simulink model "PX4_Run_Mode_R2016b"  (R2017b)
settings: Solver=FixedStepDiscrete  StartTime=0.0  StopTime=inf  FixedStep=Ts  RelTol=1e-3  EnableMultiTasking=on
InitFcn:
  | run('InitFcn_R2016b.m');
values from neighbouring files (symbols this model uses):
  A = Pixhawk_CSC.Parameter( {single([diag([1 1 1]) Ts*diag([1 1 1]); diag([0 0 0]) diag([1 1 1])]),'A'} )    [InitFcn.m]    (also in InitFcn_R2016b.m; InitFcn_R2017b_no_csc.m = single([diag([1 1 1]) Ts*diag([1 1 1]); diag([0 0 0]) diag([)
  app = Pixhawk_CSC.Parameter({single( [0.05; 0.05; 0.05]),'app'} )    [InitFcn.m]    (also in InitFcn_R2016b.m; InitFcn_R2017b_no_csc.m = single( [0.05; 0.05; 0.05]))
  B = Pixhawk_CSC.Parameter( {single([Ts^2/2*diag([1 1 1]); Ts*diag([1 1 1])]),'B'} )    [InitFcn.m]    (also in InitFcn_R2016b.m; InitFcn_R2017b_no_csc.m = single([Ts^2/2*diag([1 1 1]); Ts*diag([1 1 1])]))
  Beta = Pixhawk_CSC.Parameter({single( 0.02),'Beta'} )    [InitFcn.m]    (also in InitFcn_R2016b.m; InitFcn_R2017b_no_csc.m = single( 0.02))
  C = Pixhawk_CSC.Parameter( {single([diag([1 1 1]) 0*diag([1 1 1]); zeros(1,2) 1 zeros(1,3)]),'C'} )    [InitFcn.m]    (also in InitFcn_R2016b.m; InitFcn_R2017b_no_csc.m = single([diag([1 1 1]) 0*diag([1 1 1]); zeros(1,2) 1 zeros(1,)
  C1 = Pixhawk_CSC.Parameter({single( 1.08680),'C1'} )    [InitFcn.m]    (also in InitFcn_R2016b.m; InitFcn_R2017b_no_csc.m = single( 1.08680))
  C10 = Pixhawk_CSC.Parameter({single( 0.0000),'C10'} )    [InitFcn.m]    (also in InitFcn_R2016b.m; InitFcn_R2017b_no_csc.m = single( 0.0000))
  C11 = Pixhawk_CSC.Parameter({single(-0.2300),'C11'} )    [InitFcn.m]    (also in InitFcn_R2016b.m; InitFcn_R2017b_no_csc.m = single(-0.2300))
  C12 = Pixhawk_CSC.Parameter({single( 0.0000),'C12'} )    [InitFcn.m]    (also in InitFcn_R2016b.m; InitFcn_R2017b_no_csc.m = single( 0.0000))
  C13 = Pixhawk_CSC.Parameter({single( 0.8000),'C13'} )    [InitFcn.m]    (also in InitFcn_R2016b.m; InitFcn_R2017b_no_csc.m = single( 0.8000))
  C14 = Pixhawk_CSC.Parameter({single( 0.8000),'C14'} )    [InitFcn.m]    (also in InitFcn_R2016b.m; InitFcn_R2017b_no_csc.m = single( 0.8000))
  C15 = Pixhawk_CSC.Parameter({single( 1.73200),'C15'} )    [InitFcn.m]    (also in InitFcn_R2016b.m; InitFcn_R2017b_no_csc.m = single( 1.73200))
  C16 = Pixhawk_CSC.Parameter({single( 0.1000),'C16'} )    [InitFcn.m]    (also in InitFcn_R2016b.m; InitFcn_R2017b_no_csc.m = single( 0.1000))
  C17 = Pixhawk_CSC.Parameter({single( 0.1000),'C17'} )    [InitFcn.m]    (also in InitFcn_R2016b.m; InitFcn_R2017b_no_csc.m = single( 0.1000))
  C18 = Pixhawk_CSC.Parameter({single( 0.0500),'C18'} )    [InitFcn.m]    (also in InitFcn_R2016b.m; InitFcn_R2017b_no_csc.m = single( 0.0500))
  C19 = Pixhawk_CSC.Parameter({single( 0.6000),'C19'} )    [InitFcn.m]    (also in InitFcn_R2016b.m; InitFcn_R2017b_no_csc.m = single( 0.6000))
  C2 = Pixhawk_CSC.Parameter({single( 1.10468),'C2'} )    [InitFcn.m]    (also in InitFcn_R2016b.m; InitFcn_R2017b_no_csc.m = single( 1.10468))
  C20 = Pixhawk_CSC.Parameter({single( 0.6000),'C20'} )    [InitFcn.m]    (also in InitFcn_R2016b.m; InitFcn_R2017b_no_csc.m = single( 0.6000))
  C21 = Pixhawk_CSC.Parameter({single( 1.04558),'C21'} )    [InitFcn.m]    (also in InitFcn_R2016b.m; InitFcn_R2017b_no_csc.m = single( 1.04558))
  C22 = Pixhawk_CSC.Parameter({single( 0.0000),'C22'} )    [InitFcn.m]    (also in InitFcn_R2016b.m; InitFcn_R2017b_no_csc.m = single( 0.0000))
  C23 = Pixhawk_CSC.Parameter({single( 0.0000),'C23'} )    [InitFcn.m]    (also in InitFcn_R2016b.m; InitFcn_R2017b_no_csc.m = single( 0.0000))
  C24 = Pixhawk_CSC.Parameter({single(-11.0000),'C24'} )    [InitFcn.m]    (also in InitFcn_R2016b.m; InitFcn_R2017b_no_csc.m = single(-11.0000))
  C3 = Pixhawk_CSC.Parameter({single( 1.1980),'C3'} )    [InitFcn.m]    (also in InitFcn_R2016b.m; InitFcn_R2017b_no_csc.m = single( 1.1980))
  C4 = Pixhawk_CSC.Parameter({single( 0.0500),'C4'} )    [InitFcn.m]    (also in InitFcn_R2016b.m; InitFcn_R2017b_no_csc.m = single( 0.0500))
  C5 = Pixhawk_CSC.Parameter({single( 0.0500),'C5'} )    [InitFcn.m]    (also in InitFcn_R2016b.m; InitFcn_R2017b_no_csc.m = single( 0.0500))
  C6 = Pixhawk_CSC.Parameter({single( 0.0500),'C6'} )    [InitFcn.m]    (also in InitFcn_R2016b.m; InitFcn_R2017b_no_csc.m = single( 0.0500))
  C7 = Pixhawk_CSC.Parameter({single( 0.35937),'C7'} )    [InitFcn.m]    (also in InitFcn_R2016b.m; InitFcn_R2017b_no_csc.m = single( 0.35937))
  C8 = Pixhawk_CSC.Parameter({single( 0.36528),'C8'} )    [InitFcn.m]    (also in InitFcn_R2016b.m; InitFcn_R2017b_no_csc.m = single( 0.36528))
  C9 = Pixhawk_CSC.Parameter({single( 0.53311),'C9'} )    [InitFcn.m]    (also in InitFcn_R2016b.m; InitFcn_R2017b_no_csc.m = single( 0.53311))
  C_1 = Pixhawk_CSC.Parameter( {single([diag([1 1 1]) 0*diag([1 1 1])]),'C1'} )    [InitFcn.m]    (also in InitFcn_R2016b.m; InitFcn_R2017b_no_csc.m = single([diag([1 1 1]) 0*diag([1 1 1])]))
  CAL_ACC0_XOFFSET = Pixhawk_CSC.Parameter( {single( 0.122052  ),'CAL_ACC0_XOFFSET'} )    [InitFcn.m]    (also in InitFcn_R2016b.m; InitFcn_R2017b_no_csc.m = single( 0.122052  ))
  CAL_ACC0_XXSCALE = Pixhawk_CSC.Parameter( {single(  1.01218    ),'CAL_ACC0_XXSCALE'} )    [InitFcn.m]    (also in InitFcn_R2016b.m; InitFcn_R2017b_no_csc.m = single(  1.01218    ))
  CAL_ACC0_XYSCALE = Pixhawk_CSC.Parameter( {single( -0.00443301 ),'CAL_ACC0_XYSCALE'} )    [InitFcn.m]    (also in InitFcn_R2016b.m; InitFcn_R2017b_no_csc.m = single( -0.00443301 ))
  CAL_ACC0_XZSCALE = Pixhawk_CSC.Parameter( {single( -0.00505793 ),'CAL_ACC0_XZSCALE'} )    [InitFcn.m]    (also in InitFcn_R2016b.m; InitFcn_R2017b_no_csc.m = single( -0.00505793 ))
  CAL_ACC0_YOFFSET = Pixhawk_CSC.Parameter( {single( 0.00281205),'CAL_ACC0_YOFFSET'} )    [InitFcn.m]    (also in InitFcn_R2016b.m; InitFcn_R2017b_no_csc.m = single( 0.00281205))
  CAL_ACC0_YXSCALE = Pixhawk_CSC.Parameter( {single( -0.00443301 ),'CAL_ACC0_YXSCALE'} )    [InitFcn.m]    (also in InitFcn_R2016b.m; InitFcn_R2017b_no_csc.m = single( -0.00443301 ))
  CAL_ACC0_YYSCALE = Pixhawk_CSC.Parameter( {single(  1.00234    ),'CAL_ACC0_YYSCALE'} )    [InitFcn.m]    (also in InitFcn_R2016b.m; InitFcn_R2017b_no_csc.m = single(  1.00234    ))
  CAL_ACC0_YZSCALE = Pixhawk_CSC.Parameter( {single(  0.0160883  ),'CAL_ACC0_YZSCALE'} )    [InitFcn.m]    (also in InitFcn_R2016b.m; InitFcn_R2017b_no_csc.m = single(  0.0160883  ))
  CAL_ACC0_ZOFFSET = Pixhawk_CSC.Parameter( {single(-0.0298121 ),'CAL_ACC0_ZOFFSET'} )    [InitFcn.m]    (also in InitFcn_R2016b.m; InitFcn_R2017b_no_csc.m = single(-0.0298121 ))
  CAL_ACC0_ZXSCALE = Pixhawk_CSC.Parameter( {single( -0.00505793 ),'CAL_ACC0_ZXSCALE'} )    [InitFcn.m]    (also in InitFcn_R2016b.m; InitFcn_R2017b_no_csc.m = single( -0.00505793 ))
  CAL_ACC0_ZYSCALE = Pixhawk_CSC.Parameter( {single(  0.0160883  ),'CAL_ACC0_ZYSCALE'} )    [InitFcn.m]    (also in InitFcn_R2016b.m; InitFcn_R2017b_no_csc.m = single(  0.0160883  ))
  CAL_ACC0_ZZSCALE = Pixhawk_CSC.Parameter( {single(  0.983604   ),'CAL_ACC0_ZZSCALE'} )    [InitFcn.m]    (also in InitFcn_R2016b.m; InitFcn_R2017b_no_csc.m = single(  0.983604   ))
  CAL_BAR_OFFSET = Pixhawk_CSC.Parameter( {single( -20.8468),'CAL_BAR_OFFSET'} )    [InitFcn.m]    (also in InitFcn_R2016b.m; InitFcn_R2017b_no_csc.m = single( -20.8468))
  CAL_BAR_SCALE = Pixhawk_CSC.Parameter( {single(   1.0632),'CAL_BAR_SCALE'} )    [InitFcn.m]    (also in InitFcn_R2016b.m; InitFcn_R2017b_no_csc.m = single(   1.0632))
  CAL_BAT0_XOFFSET = Pixhawk_CSC.Parameter( {single( 0.0000),'CAL_BAT0_XOFFSET'} )    [InitFcn.m]    (also in InitFcn_R2016b.m; InitFcn_R2017b_no_csc.m = single( 0.0000))
  CAL_BAT0_XXSCALE = Pixhawk_CSC.Parameter( {single(  1.0000),'CAL_BAT0_XXSCALE'} )    [InitFcn.m]    (also in InitFcn_R2016b.m; InitFcn_R2017b_no_csc.m = single(  1.0000))
  CAL_BAT0_XYSCALE = Pixhawk_CSC.Parameter( {single(  0.0000),'CAL_BAT0_XYSCALE'} )    [InitFcn.m]    (also in InitFcn_R2016b.m; InitFcn_R2017b_no_csc.m = single(  0.0000))
  CAL_BAT0_XZSCALE = Pixhawk_CSC.Parameter( {single(  0.0000),'CAL_BAT0_XZSCALE'} )    [InitFcn.m]    (also in InitFcn_R2016b.m; InitFcn_R2017b_no_csc.m = single(  0.0000))
  CAL_BAT0_YOFFSET = Pixhawk_CSC.Parameter( {single( 0.0000),'CAL_BAT0_YOFFSET'} )    [InitFcn.m]    (also in InitFcn_R2016b.m; InitFcn_R2017b_no_csc.m = single( 0.0000))
  CAL_BAT0_YXSCALE = Pixhawk_CSC.Parameter( {single(  0.0000),'CAL_BAT0_YXSCALE'} )    [InitFcn.m]    (also in InitFcn_R2016b.m; InitFcn_R2017b_no_csc.m = single(  0.0000))
  CAL_BAT0_YYSCALE = Pixhawk_CSC.Parameter( {single(  1.0000),'CAL_BAT0_YYSCALE'} )    [InitFcn.m]    (also in InitFcn_R2016b.m; InitFcn_R2017b_no_csc.m = single(  1.0000))
  CAL_BAT0_YZSCALE = Pixhawk_CSC.Parameter( {single(  0.0000),'CAL_BAT0_YZSCALE'} )    [InitFcn.m]    (also in InitFcn_R2016b.m; InitFcn_R2017b_no_csc.m = single(  0.0000))
  CAL_BAT0_ZOFFSET = Pixhawk_CSC.Parameter( {single( 0.0000),'CAL_BAT0_ZOFFSET'} )    [InitFcn.m]    (also in InitFcn_R2016b.m; InitFcn_R2017b_no_csc.m = single( 0.0000))
  CAL_BAT0_ZXSCALE = Pixhawk_CSC.Parameter( {single(  0.0000),'CAL_BAT0_ZXSCALE'} )    [InitFcn.m]    (also in InitFcn_R2016b.m; InitFcn_R2017b_no_csc.m = single(  0.0000))
  CAL_BAT0_ZYSCALE = Pixhawk_CSC.Parameter( {single(  0.0000),'CAL_BAT0_ZYSCALE'} )    [InitFcn.m]    (also in InitFcn_R2016b.m; InitFcn_R2017b_no_csc.m = single(  0.0000))
  CAL_BAT0_ZZSCALE = Pixhawk_CSC.Parameter( {single(  1.0000),'CAL_BAT0_ZZSCALE'} )    [InitFcn.m]    (also in InitFcn_R2016b.m; InitFcn_R2017b_no_csc.m = single(  1.0000))
  CAL_GPS0_XOFFSET = Pixhawk_CSC.Parameter( {single( 0.0000),'CAL_GPS0_XOFFSET'} )    [InitFcn.m]    (also in InitFcn_R2016b.m; InitFcn_R2017b_no_csc.m = single( 0.0000))
  CAL_GPS0_XXSCALE = Pixhawk_CSC.Parameter( {single(  0.0100),'CAL_GPS0_XXSCALE'} )    [InitFcn.m]    (also in InitFcn_R2016b.m; InitFcn_R2017b_no_csc.m = single(  0.0100))
  CAL_GPS0_XYSCALE = Pixhawk_CSC.Parameter( {single(  0.0000),'CAL_GPS0_XYSCALE'} )    [InitFcn.m]    (also in InitFcn_R2016b.m; InitFcn_R2017b_no_csc.m = single(  0.0000))
  CAL_GPS0_XZSCALE = Pixhawk_CSC.Parameter( {single(  0.0000),'CAL_GPS0_XZSCALE'} )    [InitFcn.m]    (also in InitFcn_R2016b.m; InitFcn_R2017b_no_csc.m = single(  0.0000))
  CAL_GPS0_YOFFSET = Pixhawk_CSC.Parameter( {single( 0.0000),'CAL_GPS0_YOFFSET'} )    [InitFcn.m]    (also in InitFcn_R2016b.m; InitFcn_R2017b_no_csc.m = single( 0.0000))
  CAL_GPS0_YXSCALE = Pixhawk_CSC.Parameter( {single(  0.0000),'CAL_GPS0_YXSCALE'} )    [InitFcn.m]    (also in InitFcn_R2016b.m; InitFcn_R2017b_no_csc.m = single(  0.0000))
  CAL_GPS0_YYSCALE = Pixhawk_CSC.Parameter( {single(  0.0100),'CAL_GPS0_YYSCALE'} )    [InitFcn.m]    (also in InitFcn_R2016b.m; InitFcn_R2017b_no_csc.m = single(  0.0100))
  CAL_GPS0_YZSCALE = Pixhawk_CSC.Parameter( {single(  0.0000),'CAL_GPS0_YZSCALE'} )    [InitFcn.m]    (also in InitFcn_R2016b.m; InitFcn_R2017b_no_csc.m = single(  0.0000))
  CAL_GPS0_ZOFFSET = Pixhawk_CSC.Parameter( {single( 0.0000),'CAL_GPS0_ZOFFSET'} )    [InitFcn.m]    (also in InitFcn_R2016b.m; InitFcn_R2017b_no_csc.m = single( 0.0000))
  CAL_GPS0_ZXSCALE = Pixhawk_CSC.Parameter( {single(  0.0000),'CAL_GPS0_ZXSCALE'} )    [InitFcn.m]    (also in InitFcn_R2016b.m; InitFcn_R2017b_no_csc.m = single(  0.0000))
  CAL_GPS0_ZYSCALE = Pixhawk_CSC.Parameter( {single(  0.0000),'CAL_GPS0_ZYSCALE'} )    [InitFcn.m]    (also in InitFcn_R2016b.m; InitFcn_R2017b_no_csc.m = single(  0.0000))
  CAL_GPS0_ZZSCALE = Pixhawk_CSC.Parameter( {single( -0.0010),'CAL_GPS0_ZZSCALE'} )    [InitFcn.m]    (also in InitFcn_R2016b.m; InitFcn_R2017b_no_csc.m = single( -0.0010))
  CAL_GYRO0_XXSCALE = Pixhawk_CSC.Parameter( {single(0.992736),'CAL_GYRO0_XXSCALE'} )    [InitFcn.m]    (also in InitFcn_R2016b.m; InitFcn_R2017b_no_csc.m = single(0.992736))
  CAL_GYRO0_XYSCALE = Pixhawk_CSC.Parameter( {single(0.0000),'CAL_GYRO0_XYSCALE'} )    [InitFcn.m]    (also in InitFcn_R2016b.m; InitFcn_R2017b_no_csc.m = single(0.0000))
  CAL_GYRO0_XZSCALE = Pixhawk_CSC.Parameter( {single(0.0000),'CAL_GYRO0_XZSCALE'} )    [InitFcn.m]    (also in InitFcn_R2016b.m; InitFcn_R2017b_no_csc.m = single(0.0000))
  CAL_GYRO0_YXSCALE = Pixhawk_CSC.Parameter( {single(0.0000),'CAL_GYRO0_YXSCALE'} )    [InitFcn.m]    (also in InitFcn_R2016b.m; InitFcn_R2017b_no_csc.m = single(0.0000))
  CAL_GYRO0_YYSCALE = Pixhawk_CSC.Parameter( {single(1.01609),'CAL_GYRO0_YYSCALE'} )    [InitFcn.m]    (also in InitFcn_R2016b.m; InitFcn_R2017b_no_csc.m = single(1.01609))
  CAL_GYRO0_YZSCALE = Pixhawk_CSC.Parameter( {single(0.0000),'CAL_GYRO0_YZSCALE'} )    [InitFcn.m]    (also in InitFcn_R2016b.m; InitFcn_R2017b_no_csc.m = single(0.0000))
  CAL_GYRO0_ZXSCALE = Pixhawk_CSC.Parameter( {single(0.0000),'CAL_GYRO0_ZXSCALE'} )    [InitFcn.m]    (also in InitFcn_R2016b.m; InitFcn_R2017b_no_csc.m = single(0.0000))
  CAL_GYRO0_ZYSCALE = Pixhawk_CSC.Parameter( {single(0.0000),'CAL_GYRO0_ZYSCALE'} )    [InitFcn.m]    (also in InitFcn_R2016b.m; InitFcn_R2017b_no_csc.m = single(0.0000))
  CAL_GYRO0_ZZSCALE = Pixhawk_CSC.Parameter( {single(1.03003),'CAL_GYRO0_ZZSCALE'} )    [InitFcn.m]    (also in InitFcn_R2016b.m; InitFcn_R2017b_no_csc.m = single(1.03003))
  CAL_MAG0_XCURCOR = Pixhawk_CSC.Parameter( {single( 0.0017     ),'CAL_MAG0_XCURCOR'} )    [InitFcn.m]    (also in InitFcn_R2016b.m; InitFcn_R2017b_no_csc.m = single( 0.0017     ))
  CAL_MAG0_XOFFSET = Pixhawk_CSC.Parameter( {single( 0.0446372  ),'CAL_MAG0_XOFFSET'} )    [InitFcn.m]    (also in InitFcn_R2016b.m; InitFcn_R2017b_no_csc.m = single( 0.0446372  ))
  CAL_MAG0_XXSCALE = Pixhawk_CSC.Parameter( {single(  1.01563   ),'CAL_MAG0_XXSCALE'} )    [InitFcn.m]    (also in InitFcn_R2016b.m; InitFcn_R2017b_no_csc.m = single(  1.01563   ))
  CAL_MAG0_XYSCALE = Pixhawk_CSC.Parameter( {single( -0.0612061 ),'CAL_MAG0_XYSCALE'} )    [InitFcn.m]    (also in InitFcn_R2016b.m; InitFcn_R2017b_no_csc.m = single( -0.0612061 ))
  CAL_MAG0_XZSCALE = Pixhawk_CSC.Parameter( {single( -0.011532  ),'CAL_MAG0_XZSCALE'} )    [InitFcn.m]    (also in InitFcn_R2016b.m; InitFcn_R2017b_no_csc.m = single( -0.011532  ))
  CAL_MAG0_YCURCOR = Pixhawk_CSC.Parameter( {single(-0.0075     ),'CAL_MAG0_YCURCOR'} )    [InitFcn.m]    (also in InitFcn_R2016b.m; InitFcn_R2017b_no_csc.m = single(-0.0075     ))
  CAL_MAG0_YOFFSET = Pixhawk_CSC.Parameter( {single( 0.0700776  ),'CAL_MAG0_YOFFSET'} )    [InitFcn.m]    (also in InitFcn_R2016b.m; InitFcn_R2017b_no_csc.m = single( 0.0700776  ))
  CAL_MAG0_YXSCALE = Pixhawk_CSC.Parameter( {single( -0.0612061 ),'CAL_MAG0_YXSCALE'} )    [InitFcn.m]    (also in InitFcn_R2016b.m; InitFcn_R2017b_no_csc.m = single( -0.0612061 ))
  CAL_MAG0_YYSCALE = Pixhawk_CSC.Parameter( {single(  1.00593   ),'CAL_MAG0_YYSCALE'} )    [InitFcn.m]    (also in InitFcn_R2016b.m; InitFcn_R2017b_no_csc.m = single(  1.00593   ))
  CAL_MAG0_YZSCALE = Pixhawk_CSC.Parameter( {single(  0.0144582 ),'CAL_MAG0_YZSCALE'} )    [InitFcn.m]    (also in InitFcn_R2016b.m; InitFcn_R2017b_no_csc.m = single(  0.0144582 ))
  CAL_MAG0_ZCURCOR = Pixhawk_CSC.Parameter( {single(-0.0080     ),'CAL_MAG0_ZCURCOR'} )    [InitFcn.m]    (also in InitFcn_R2016b.m; InitFcn_R2017b_no_csc.m = single(-0.0080     ))
  CAL_MAG0_ZOFFSET = Pixhawk_CSC.Parameter( {single( 0.00201742 ),'CAL_MAG0_ZOFFSET'} )    [InitFcn.m]    (also in InitFcn_R2016b.m; InitFcn_R2017b_no_csc.m = single( 0.00201742 ))
  CAL_MAG0_ZXSCALE = Pixhawk_CSC.Parameter( {single( -0.011532  ),'CAL_MAG0_ZXSCALE'} )    [InitFcn.m]    (also in InitFcn_R2016b.m; InitFcn_R2017b_no_csc.m = single( -0.011532  ))
  CAL_MAG0_ZYSCALE = Pixhawk_CSC.Parameter( {single(  0.0144582 ),'CAL_MAG0_ZYSCALE'} )    [InitFcn.m]    (also in InitFcn_R2016b.m; InitFcn_R2017b_no_csc.m = single(  0.0144582 ))
  CAL_MAG0_ZZSCALE = Pixhawk_CSC.Parameter( {single(  0.986813  ),'CAL_MAG0_ZZSCALE'} )    [InitFcn.m]    (also in InitFcn_R2016b.m; InitFcn_R2017b_no_csc.m = single(  0.986813  ))
  CAL_SONAR_OFFSET = Pixhawk_CSC.Parameter( {single( -6.8730),'CAL_SONAR_OFFSET'} )    [InitFcn.m]    (also in InitFcn_R2016b.m; InitFcn_R2017b_no_csc.m = single( -6.8730))
  CAL_SONAR_SCALE = Pixhawk_CSC.Parameter( {single(-438.1875),'CAL_SONAR_SCALE'} )    [InitFcn.m]    (also in InitFcn_R2016b.m; InitFcn_R2017b_no_csc.m = single(-438.1875))
  COM_RATE = double(10)    [InitFcn.m]    (also in InitFcn_R2016b.m; InitFcn_R2017b_no_csc.m)
  D = Pixhawk_CSC.Parameter( {single(zeros(size(C.Value,1), size(B.Value,2))),'D'} )    [InitFcn.m]    (also in InitFcn_R2016b.m; InitFcn_R2017b_no_csc.m = single(zeros(size(C,1), size(B,2))))
  Dip0 = Pixhawk_CSC.Parameter({single( 1.2),'Dip0'} )    [InitFcn.m]    (also in InitFcn_R2016b.m; InitFcn_R2017b_no_csc.m = single( 1.2))
  I = Pixhawk_CSC.Parameter( {single(eye(size(Q.Value))),'I'} )    [InitFcn.m]    (also in InitFcn_R2016b.m; InitFcn_R2017b_no_csc.m = single(eye(size(Q))))
  Jxx = Pixhawk_CSC.Parameter( {single(J(1,1)),'Jxx'} )    [InitFcn.m]    (also in InitFcn_R2016b.m; InitFcn_R2017b_no_csc.m = single(J(1,1)))
  Jyy = Pixhawk_CSC.Parameter( {single(J(2,2)),'Jyy'} )    [InitFcn.m]    (also in InitFcn_R2016b.m; InitFcn_R2017b_no_csc.m = single(J(2,2)))
  Jzz = Pixhawk_CSC.Parameter( {single(J(3,3)),'Jzz'} )    [InitFcn.m]    (also in InitFcn_R2016b.m; InitFcn_R2017b_no_csc.m = single(J(3,3)))
  Kapp = Pixhawk_CSC.Parameter({single( 1.2),'Kapp'} )    [InitFcn.m]    (also in InitFcn_R2016b.m; InitFcn_R2017b_no_csc.m = single( 1.2))
  Kx = Pixhawk_CSC.Parameter({single( Kx),'Kx'} )    [InitFcn.m]    (also in InitFcn_R2016b.m = Pixhawk_CSC.Parameter({single( [0.60 0.9]),'Kx'} ); InitFcn_R2017b_no_csc.m = single( [0.60 0.9]))
  Ky = Pixhawk_CSC.Parameter({single( Ky),'Ky'} )    [InitFcn.m]    (also in InitFcn_R2016b.m = Pixhawk_CSC.Parameter({single( [0.4 0.9]),'Ky'} ); InitFcn_R2017b_no_csc.m = single( [0.4 0.9]))
  LPF_REF_DEN = Pixhawk_CSC.Parameter( {single([1.0000 -0.8187]),'LPF_REF_DEN'} )    [InitFcn.m]    (also in InitFcn_R2016b.m; InitFcn_R2017b_no_csc.m = single([1.0000 -0.8187]))
  LPF_REF_NUM = Pixhawk_CSC.Parameter( {single([0.0000  0.1813]),'LPF_REF_NUM'} )    [InitFcn.m]    (also in InitFcn_R2016b.m; InitFcn_R2017b_no_csc.m = single([0.0000  0.1813]))
  m0 = Pixhawk_CSC.Parameter({single( 0.452857),'m0'} )    [InitFcn.m]    (also in InitFcn_R2016b.m; InitFcn_R2017b_no_csc.m = single( 0.452857))
  mn = [0.01; 0.01; 0.01; 0.01]    [InitFcn.m]    (also in InitFcn_R2016b.m; InitFcn_R2017b_no_csc.m)
  MOV_AVG_WINDOW = Pixhawk_CSC.Parameter( {single(100),'MOV_AVG_WINDOW'} )    [InitFcn.m]    (also in InitFcn_R2016b.m; InitFcn_R2017b_no_csc.m = single(100))
  Ox0 = Pixhawk_CSC.Parameter({single(O_x0),'Ox0'} )    [InitFcn.m]    (also in InitFcn_R2016b.m; InitFcn_R2017b_no_csc.m = single(O_x0))
  Oxa = Pixhawk_CSC.Parameter({single(O_x.a),'Oxa'} )    [InitFcn.m]    (also in InitFcn_R2016b.m; InitFcn_R2017b_no_csc.m = single(O_x.a))
  Oxb = Pixhawk_CSC.Parameter({single(O_x.b),'Oxb'} )    [InitFcn.m]    (also in InitFcn_R2016b.m; InitFcn_R2017b_no_csc.m = single(O_x.b))
  Oxc = Pixhawk_CSC.Parameter({single(O_x.c),'Oxc'} )    [InitFcn.m]    (also in InitFcn_R2016b.m; InitFcn_R2017b_no_csc.m = single(O_x.c))
  Oxd = Pixhawk_CSC.Parameter({single(O_x.d),'Oxd'} )    [InitFcn.m]    (also in InitFcn_R2016b.m; InitFcn_R2017b_no_csc.m = single(O_x.d))
  Oy0 = Pixhawk_CSC.Parameter({single(O_y0),'Oy0'} )    [InitFcn.m]    (also in InitFcn_R2016b.m; InitFcn_R2017b_no_csc.m = single(O_y0))
  Oya = Pixhawk_CSC.Parameter({single(O_y.a),'Oya'} )    [InitFcn.m]    (also in InitFcn_R2016b.m; InitFcn_R2017b_no_csc.m = single(O_y.a))
  Oyb = Pixhawk_CSC.Parameter({single(O_y.b),'Oyb'} )    [InitFcn.m]    (also in InitFcn_R2016b.m; InitFcn_R2017b_no_csc.m = single(O_y.b))
  Oyc = Pixhawk_CSC.Parameter({single(O_y.c),'Oyc'} )    [InitFcn.m]    (also in InitFcn_R2016b.m; InitFcn_R2017b_no_csc.m = single(O_y.c))
  Oyd = Pixhawk_CSC.Parameter({single(O_y.d),'Oyd'} )    [InitFcn.m]    (also in InitFcn_R2016b.m; InitFcn_R2017b_no_csc.m = single(O_y.d))
  Oz0 = Pixhawk_CSC.Parameter({single(O_z0),'Oz0'} )    [InitFcn.m]    (also in InitFcn_R2016b.m; InitFcn_R2017b_no_csc.m = single(O_z0))
  ... (+53 more)
undefined symbols (not defined in the file or in its folder): AccX, AccY, AccZ, Altitude, ax, ay, az, Current, FILTER_N, GPS_TS, GyroX, GyroY, GyroZ, Latitude, Longitude, M1_PWM, M2_PWM, M3_PWM, M4_PWM, MagX, MagY, MagZ, mAH, MOTOR, phi, Position_TS, psi, PX4_TUNE_ENUM, RGBLED_COLOR_ENUM, RGBLED_MODE_ENUM, S_AccX, S_AccY, S_AccZ, S_Altitude, S_Baro, S_Current, S_GyroX, S_GyroY, S_GyroZ, S_Latitude, S_Longitude, S_MagX, S_MagY, S_MagZ, S_mAH, S_N_Sat, S_Voltage, T_PITCH, T_ROLL, T_THROTTLE, theta, v, Voltage, w, wx, wxd, wy, wyd, wz ... (+4)
libraries: simulink x31, pixhawk_slib_sensors_actuators x7, pixhawk_slib_ADC_serial x5, pixhawk_slib_misc_utils x3, etargetslib x2
(part 3 of 7)

== system PX4_Run_Mode_R2016b/SENSOR_FILTER/Bias Removal State ==
  ESTIMATED_STATE_IN : Inport
  PARAMETERS_IN : Inport  Port=2
  SYSTEM_MODE_IN : Inport  Port=3
  Bus Assignment1 : BusAssignment  AssignedSignals=State Bias Parameters.X_BIAS,State Bias Parameters.Y_BIAS,State Bias Parameters.Z_BIAS,State Bias Parameters.PHI_BIAS,State Bias Parameters.THETA_BIAS,State Bias Parameters.PSI_BIAS,State Bias Parameters.U_BIAS,State Bias Parameters.V_BIAS,State Bias Parameters.W_BIAS,State Bias Parameters.WX_BIAS,State Bias Parameters.WY_BIAS,State Bias Parameters.WZ_BIAS,State Bias Parameters.AX_BIAS,State Bias Parameters.AY_BIAS,State Bias Parameters.AZ_BIAS,State Bias Parameters.WXD_BIAS,State Bias Parameters.WYD_BIAS,State Bias Parameters.WZD_BIAS
  Bus Assignment2 : BusAssignment  AssignedSignals=x,y,z,phi,theta,psi,u,v,w,wx,wy,wz,ax,ay,az,wxd,wyd,wzd
  Bus Selector1 : BusSelector  OutputSignals=ARM_CMD,PRE_ARM_CMD
  Bus Selector4 : BusSelector  OutputSignals=x,y,z,phi,theta,psi,u,v,w,wx,wy,wz,ax,ay,az,wxd,wyd,wzd  OutputAsBus=on
  Bus to Vector : BusToVector
  Demux1 : Demux  Outputs=18
  Demux2 : Demux  Outputs=18
  Logical Operator1 : Logic  IconShape=distinctive  AllPortsSameDT=off  OutDataTypeStr=boolean
  Logical Operator2 : Logic  Operator=NOT  IconShape=distinctive  AllPortsSameDT=off  OutDataTypeStr=boolean
  Logical Operator4 : Logic  Operator=NOT  IconShape=distinctive  AllPortsSameDT=off  OutDataTypeStr=boolean
  Logical Operator5 : Logic  IconShape=distinctive  AllPortsSameDT=off  OutDataTypeStr=boolean
  MATLAB Function3 : MATLAB Function  TreatAsAtomicUnit=on
  ESTIMATED_STATE_OUT : Outport
  PARAMETERS_OUT : Outport  Port=2
  wires:
  Bus to Vector/1 -> MATLAB Function3/1(STATE_IN)
  Bus Assignment2/1 -> ESTIMATED_STATE_OUT/1
  MATLAB Function3/1(STATE_OUT) -> Demux1/1
  ESTIMATED_STATE_IN/1 -> Bus Selector4/1, Bus Assignment2/1
  Bus Selector4/1 -> Bus to Vector/1
  SYSTEM_MODE_IN/1 -> Bus Selector1/1
  Bus Selector1/1 -> Logical Operator2/1  "<ARM_CMD>"
  Logical Operator2/1 -> Logical Operator1/1, Logical Operator5/1
  Bus Selector1/2 -> Logical Operator1/2, Logical Operator4/1  "<PRE_ARM_CMD>"
  Logical Operator5/1 -> MATLAB Function3/2(RESET)
  Logical Operator4/1 -> Logical Operator5/2
  Demux1/2 -> Bus Assignment2/3
  Demux1/1 -> Bus Assignment2/2
  Demux1/3 -> Bus Assignment2/4
  Demux1/7 -> Bus Assignment2/8
  Demux1/8 -> Bus Assignment2/9
  Demux1/9 -> Bus Assignment2/10
  Demux1/10 -> Bus Assignment2/11
  Demux1/11 -> Bus Assignment2/12
  Demux1/12 -> Bus Assignment2/13
  Demux1/13 -> Bus Assignment2/14
  Demux1/14 -> Bus Assignment2/15
  Demux1/15 -> Bus Assignment2/16
  Demux1/16 -> Bus Assignment2/17
  Demux1/17 -> Bus Assignment2/18
  Demux1/18 -> Bus Assignment2/19
  MATLAB Function3/2(BIAS_STATE) -> Demux2/1
  Demux2/18 -> Bus Assignment1/19
  Demux2/17 -> Bus Assignment1/18
  Demux2/16 -> Bus Assignment1/17
  Demux2/15 -> Bus Assignment1/16
  Demux2/14 -> Bus Assignment1/15
  Demux2/13 -> Bus Assignment1/14
  Demux2/12 -> Bus Assignment1/13
  Demux2/11 -> Bus Assignment1/12
  Demux2/10 -> Bus Assignment1/11
  Demux2/9 -> Bus Assignment1/10
  Demux2/8 -> Bus Assignment1/9
  Demux2/7 -> Bus Assignment1/8
  Demux2/6 -> Bus Assignment1/7
  Demux2/5 -> Bus Assignment1/6
  Demux2/3 -> Bus Assignment1/4
  Demux2/2 -> Bus Assignment1/3
  Demux2/4 -> Bus Assignment1/5
  Demux2/1 -> Bus Assignment1/2
  PARAMETERS_IN/1 -> Bus Assignment1/1
  Bus Assignment1/1 -> PARAMETERS_OUT/1
  Logical Operator1/1 -> MATLAB Function3/3(CONFIG_CMD)
  Demux1/4 -> Bus Assignment2/5
  Demux1/5 -> Bus Assignment2/6
  Demux1/6 -> Bus Assignment2/7

== system PX4_Run_Mode_R2016b/SENSOR_FILTER/Fixed Bias removal and scaling ==
  FILTERED_SENSOR_DATA_IN : Inport
  RAW_SENSOR_DATA_IN : Inport  Port=2
  SYSTEM_MODE_IN : Inport  Port=3
  Accelerometer Calibration : Subsystem
  Barometer Calibration : Subsystem
  Battery Calibration : Subsystem
  GPS Calibration : Subsystem
  Gyroscope Calibration : Subsystem
  MagnetoMeter Calibration : Subsystem
  Parameter Bus Creation : Subsystem
  Sonar Calibration : Subsystem
  FILTERED_SENSOR_DATA_OUT : Outport
  PARAMETERS_OUT : Outport  Port=2
  wires:
  RAW_SENSOR_DATA_IN/1 -> MagnetoMeter Calibration/2(RAW_SENSOR_DATA_IN), Accelerometer Calibration/2(RAW_SENSOR_DATA_IN), Gyroscope Calibration/2(RAW_SENSOR_DATA_IN), Barometer Calibration/2(RAW_SENSOR_DATA_IN), GPS Calibration/2(RAW_SENSOR_DATA_IN), Sonar Calibration/2(RAW_SENSOR_DATA_IN), Battery Calibration/2(RAW_SENSOR_DATA_IN)
  FILTERED_SENSOR_DATA_IN/1 -> MagnetoMeter Calibration/1(FILTERED_SENSOR_DATA_IN)
  MagnetoMeter Calibration/2(FILTERED_SENSOR_DATA_OUT) -> Accelerometer Calibration/1(FILTERED_SENSOR_DATA_IN)
  Accelerometer Calibration/2(FILTERED_SENSOR_DATA_OUT) -> Gyroscope Calibration/1(FILTERED_SENSOR_DATA_IN)
  SYSTEM_MODE_IN/1 -> GPS Calibration/3(SYSTEM_MODE_IN), Gyroscope Calibration/3(SYSTEM_MODE_IN)
  Gyroscope Calibration/2(FILTERED_SENSOR_DATA_OUT) -> Barometer Calibration/1(FILTERED_SENSOR_DATA_IN)
  GPS Calibration/2(FILTERED_SENSOR_DATA_OUT) -> Battery Calibration/1(FILTERED_SENSOR_DATA_IN)
  Battery Calibration/2(FILTERED_SENSOR_DATA_OUT) -> Sonar Calibration/1(FILTERED_SENSOR_DATA_IN)
  MagnetoMeter Calibration/1(Parameters) -> Parameter Bus Creation/1(Parameters Magnetometer)
  Accelerometer Calibration/1(Parameters) -> Parameter Bus Creation/2(Parameters Accelerometer)
  Gyroscope Calibration/1(Parameters) -> Parameter Bus Creation/3(Parameters Gyroscope)
  GPS Calibration/1(Parameters) -> Parameter Bus Creation/5(Parameters GPS)
  Battery Calibration/1(Parameters) -> Parameter Bus Creation/6(Parameters Battery)
  Parameter Bus Creation/1(Parameters) -> PARAMETERS_OUT/1
  Sonar Calibration/2(FILTERED_SENSOR_DATA_OUT) -> FILTERED_SENSOR_DATA_OUT/1
  Sonar Calibration/1(Parameters) -> Parameter Bus Creation/7(Parameters Sonar)
  Barometer Calibration/2(FILTERED_SENSOR_DATA_OUT) -> GPS Calibration/1(FILTERED_SENSOR_DATA_IN)
  Barometer Calibration/1(Parameters) -> Parameter Bus Creation/4(Parameters Barometer)

== system PX4_Run_Mode_R2016b/SENSOR_FILTER/SensorData2States ==
  ESTIMATED_STATE_IN : Inport
  FILTERED_SENSOR_DATA_IN : Inport  Port=2
  SYSTEM_MODE : Inport  Port=3
  Rotational State Estimation : Subsystem
  Translational State Estimation : Subsystem
  ESTIMATED_STATE_OUT : Outport
  wires:
  ESTIMATED_STATE_IN/1 -> Rotational State Estimation/2(ESTIMATED_STATE_IN)
  Translational State Estimation/1(ESTIMATED_STATE_OUT) -> ESTIMATED_STATE_OUT/1
  SYSTEM_MODE/1 -> Rotational State Estimation/1(SYSTEM_MODE_IN)
  FILTERED_SENSOR_DATA_IN/1 -> Translational State Estimation/2(FILTERED_SENSOR_DATA_IN), Rotational State Estimation/3(FILTERED_SENSOR_DATA_IN)
  Rotational State Estimation/1(ESTIMATED_STATE_OUT) -> Translational State Estimation/1(ESTIMATED_STATE_IN)

== system PX4_Run_Mode_R2016b/SENSOR_FILTER/StateEstimatesInitialConditions ==
  Bus Creator : BusCreator  Inputs=18
  Bus Creator1 : BusCreator  Inputs=18
  Demux : Demux  Outputs=18
  Demux1 : Demux  Outputs=18
  Initial_Filteres_Sensor_Data : MATLAB Function  TreatAsAtomicUnit=on
  State Estimater Initial Conditions : MATLAB Function  TreatAsAtomicUnit=on
  ESTIMATED_STATE_OUT : Outport
  FILTERED_SENSOR_DATA_OUT : Outport  Port=2
  wires:
  State Estimater Initial Conditions/1(Xhat) -> Demux/1
  Demux/6 -> Bus Creator/6  "psi"
  Demux/7 -> Bus Creator/7  "u"
  Demux/5 -> Bus Creator/5  "theta"
  Demux/4 -> Bus Creator/4  "phi"
  Demux/8 -> Bus Creator/8  "v"
  Demux/3 -> Bus Creator/3  "z"
  Demux/9 -> Bus Creator/9  "w"
  Demux/2 -> Bus Creator/2  "y"
  Demux/10 -> Bus Creator/10  "wx"
  Demux/1 -> Bus Creator/1  "x"
  Demux/11 -> Bus Creator/11  "wy"
  Demux/12 -> Bus Creator/12  "wz"
  Bus Creator/1 -> ESTIMATED_STATE_OUT/1
  Demux/13 -> Bus Creator/13  "ax"
  Demux/14 -> Bus Creator/14  "ay"
  Demux/15 -> Bus Creator/15  "az"
  Demux/16 -> Bus Creator/16  "wxd"
  Demux/17 -> Bus Creator/17  "wyd"
  Demux/18 -> Bus Creator/18  "wzd"
  Initial_Filteres_Sensor_Data/1(S) -> Demux1/1
  Bus Creator1/1 -> FILTERED_SENSOR_DATA_OUT/1
  Demux1/8 -> Bus Creator1/8  "GyroY"
  Demux1/7 -> Bus Creator1/7  "GyroX"
  Demux1/9 -> Bus Creator1/9  "GyroZ"
  Demux1/6 -> Bus Creator1/6  "AccZ"
  Demux1/10 -> Bus Creator1/10  "Bar"
  Demux1/11 -> Bus Creator1/11  "Latitude"
  Demux1/5 -> Bus Creator1/5  "AccY"
  Demux1/4 -> Bus Creator1/4  "AccX"
  Demux1/12 -> Bus Creator1/12  "Longitude"
  Demux1/13 -> Bus Creator1/13  "Altitude"
  Demux1/3 -> Bus Creator1/3  "MagZ"
  Demux1/2 -> Bus Creator1/2  "MagY"
  Demux1/14 -> Bus Creator1/14  "Num_Sat"
  Demux1/15 -> Bus Creator1/15  "Voltage"
  Demux1/1 -> Bus Creator1/1  "MagX"
  Demux1/16 -> Bus Creator1/16  "Current"
  Demux1/17 -> Bus Creator1/17  "mAH"
  Demux1/18 -> Bus Creator1/18  "Sonar"

== system PX4_Run_Mode_R2016b/CONTROLLER/Inner Control Loop/Pitch Control ==
  ERROR_IN : Inport
  TARGET : Inport  Port=2
  ESTIMATED_STATE_IN : Inport  Port=3
  "SYSTEM_MODE_IN " : Inport  Port=4
  Add1 : Sum  Inputs=+-
  Add3 : Sum  Inputs=+-
  Add4 : Sum  Inputs=++++
  Bus Assignment : BusAssignment  AssignedSignals=e6,e7,e8,e9,e10
  Bus Selector1 : BusSelector  OutputSignals=ARM_CMD
  Bus Selector10 : BusSelector  OutputSignals=T_PITCH
  Bus Selector11 : BusSelector  OutputSignals=theta,wy
  Constant : Constant  Value=0  SampleTime=Ts
  Constant1 : Constant  Value=C11  SampleTime=Ts
  Data Type Conversion : DataTypeConversion  OutDataTypeStr=single
  Gain : Gain  Gain=C2
  Gain1 : Gain  Gain=C8
  Logical Operator8 : Logic  Operator=NOT  IconShape=distinctive  AllPortsSameDT=off  OutDataTypeStr=boolean
  MATLAB Function : MATLAB Function  TreatAsAtomicUnit=on
  Saturation : Saturate  UpperLimit=2  LowerLimit=-2
  U Pitch : Outport
  ERROR_OUT : Outport  Port=2
  wires:
  ESTIMATED_STATE_IN/1 -> Bus Selector11/1
  TARGET/1 -> Bus Selector10/1
  Gain1/1 -> Bus Assignment/4, Add4/3
  Gain/1 -> Add4/1, Bus Assignment/2
  Add3/1 -> Gain/1, MATLAB Function/2(u)
  Bus Selector11/1 -> Add3/2  "<theta>"
  Bus Selector10/1 -> Add3/1  "<T_PITCH>"
  Add4/1 -> Saturation/1
  ERROR_IN/1 -> Bus Assignment/1
  Bus Assignment/1 -> ERROR_OUT/1
  MATLAB Function/1(y) -> Bus Assignment/3, Add4/2
  Constant1/1 -> Bus Assignment/5, Add4/4
  "SYSTEM_MODE_IN "/1 -> Bus Selector1/1
  Bus Selector1/1 -> Logical Operator8/1  "<ARM_CMD>"
  Logical Operator8/1 -> MATLAB Function/1(Reset)
  Saturation/1 -> Bus Assignment/6, U Pitch/1
  Constant/1 -> Data Type Conversion/1
  Add1/1 -> Gain1/1
  Bus Selector11/2 -> Add1/2  "<wy>"
  Data Type Conversion/1 -> Add1/1

== system PX4_Run_Mode_R2016b/CONTROLLER/Inner Control Loop/Roll Control ==
  ERROR_IN : Inport
  TARGET : Inport  Port=2
  ESTIMATED_STATE_IN : Inport  Port=3
  "SYSTEM_MODE_IN " : Inport  Port=4
  Add1 : Sum  Inputs=+-
  Add3 : Sum  Inputs=+-
  Add4 : Sum  Inputs=++++
  Bus Assignment : BusAssignment  AssignedSignals=e1,e2,e3,e4,e5
  Bus Selector1 : BusSelector  OutputSignals=ARM_CMD
  Bus Selector10 : BusSelector  OutputSignals=T_ROLL
  Bus Selector11 : BusSelector  OutputSignals=phi,wx
  Constant : Constant  Value=0  SampleTime=Ts
  Constant1 : Constant  Value=C10
  Data Type Conversion : DataTypeConversion  OutDataTypeStr=single
  Gain : Gain  Gain=C1
  Gain1 : Gain  Gain=C7
  Logical Operator8 : Logic  Operator=NOT  IconShape=distinctive  AllPortsSameDT=off  OutDataTypeStr=boolean
  MATLAB Function : MATLAB Function  TreatAsAtomicUnit=on
  Saturation : Saturate  UpperLimit=2  LowerLimit=-2
  U Roll : Outport
  ERROR_OUT : Outport  Port=2
  wires:
  ESTIMATED_STATE_IN/1 -> Bus Selector11/1
  TARGET/1 -> Bus Selector10/1
  Add1/1 -> Gain1/1
  Gain1/1 -> Bus Assignment/4, Add4/2
  Gain/1 -> Add4/1, Bus Assignment/2
  Add3/1 -> Gain/1, MATLAB Function/2(u)
  Bus Selector11/1 -> Add3/2  "<phi>"
  Bus Selector10/1 -> Add3/1  "<T_ROLL>"
  Add4/1 -> Saturation/1
  ERROR_IN/1 -> Bus Assignment/1
  Bus Assignment/1 -> ERROR_OUT/1
  Constant1/1 -> Bus Assignment/5, Add4/3
  MATLAB Function/1(y) -> Bus Assignment/3, Add4/4
  "SYSTEM_MODE_IN "/1 -> Bus Selector1/1
  Bus Selector1/1 -> Logical Operator8/1  "<ARM_CMD>"
  Logical Operator8/1 -> MATLAB Function/1(Reset)
  Saturation/1 -> Bus Assignment/6, U Roll/1
  Bus Selector11/2 -> Add1/2  "<wx>"
  Constant/1 -> Data Type Conversion/1
  Data Type Conversion/1 -> Add1/1

== system PX4_Run_Mode_R2016b/CONTROLLER/Inner Control Loop/Yaw Control ==
  ERROR_IN : Inport
  TARGET : Inport  Port=2
  ESTIMATED_STATE_IN : Inport  Port=3
  "SYSTEM_MODE_IN " : Inport  Port=4
  Add1 : Sum  Inputs=+-
  Add3 : Sum  Inputs=+-
  Add4 : Sum  Inputs=++++
  Bus Assignment : BusAssignment  AssignedSignals=e11,e12,e13,e14,e15
  Bus Selector1 : BusSelector  OutputSignals=ARM_CMD
  Bus Selector10 : BusSelector  OutputSignals=T_YAW
  Bus Selector11 : BusSelector  OutputSignals=psi,wz
  Constant : Constant  Value=0  SampleTime=Ts
  Constant1 : Constant  Value=C12  SampleTime=Ts
  Data Type Conversion : DataTypeConversion  OutDataTypeStr=single
  Gain : Gain  Gain=C3
  Gain1 : Gain  Gain=C9
  Logical Operator8 : Logic  Operator=NOT  IconShape=distinctive  AllPortsSameDT=off  OutDataTypeStr=boolean
  MATLAB Function : MATLAB Function  TreatAsAtomicUnit=on
  Saturation : Saturate  UpperLimit=2  LowerLimit=-2
  U Yaw : Outport
  ERROR_OUT : Outport  Port=2
  wires:
  ESTIMATED_STATE_IN/1 -> Bus Selector11/1
  TARGET/1 -> Bus Selector10/1
  Gain1/1 -> Bus Assignment/4, Add4/3
  Gain/1 -> Bus Assignment/2, Add4/1
  Add3/1 -> Gain/1, MATLAB Function/2(e)
  Bus Selector10/1 -> Add3/1  "<T_YAW>"
  Add4/1 -> Saturation/1
  Bus Selector11/1 -> Add3/2  "<psi>"
  ERROR_IN/1 -> Bus Assignment/1
  Bus Assignment/1 -> ERROR_OUT/1
  Constant1/1 -> Bus Assignment/5, Add4/4
  MATLAB Function/1(eI) -> Bus Assignment/3, Add4/2
  "SYSTEM_MODE_IN "/1 -> Bus Selector1/1
  Bus Selector1/1 -> Logical Operator8/1  "<ARM_CMD>"
  Logical Operator8/1 -> MATLAB Function/1(Reset)
  Saturation/1 -> Bus Assignment/6, U Yaw/1
  Add1/1 -> Gain1/1
  Bus Selector11/2 -> Add1/2  "<wz>"
  Constant/1 -> Data Type Conversion/1
  Data Type Conversion/1 -> Add1/1

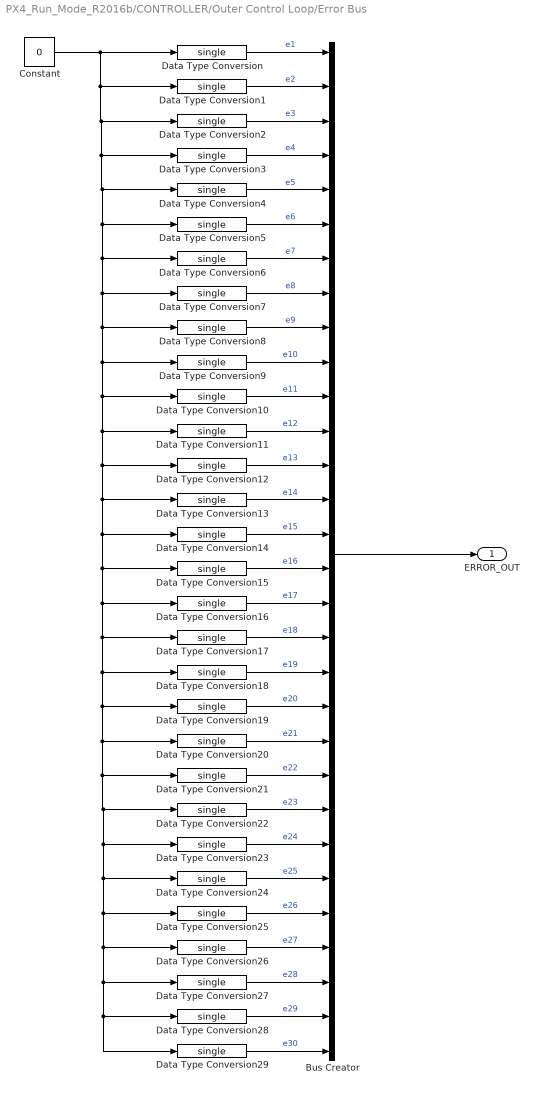
== system PX4_Run_Mode_R2016b/CONTROLLER/Outer Control Loop/Error Bus ==
  Bus Creator : BusCreator  Inputs=30
  Constant : Constant  Value=0  SampleTime=Ts
  Data Type Conversion{,1..29} (30 alike) : DataTypeConversion  OutDataTypeStr=single
  ERROR_OUT : Outport
  wires:
  Bus Creator/1 -> ERROR_OUT/1
  Data Type Conversion/1 -> Bus Creator/1  "e1"
  Data Type Conversion1/1 -> Bus Creator/2  "e2"
  Data Type Conversion2/1 -> Bus Creator/3  "e3"
  Data Type Conversion3/1 -> Bus Creator/4  "e4"
  Data Type Conversion4/1 -> Bus Creator/5  "e5"
  Data Type Conversion5/1 -> Bus Creator/6  "e6"
  Data Type Conversion6/1 -> Bus Creator/7  "e7"
  Data Type Conversion7/1 -> Bus Creator/8  "e8"
  Data Type Conversion8/1 -> Bus Creator/9  "e9"
  Data Type Conversion9/1 -> Bus Creator/10  "e10"
  Data Type Conversion10/1 -> Bus Creator/11  "e11"
  Data Type Conversion11/1 -> Bus Creator/12  "e12"
  Data Type Conversion12/1 -> Bus Creator/13  "e13"
  Data Type Conversion13/1 -> Bus Creator/14  "e14"
  Data Type Conversion14/1 -> Bus Creator/15  "e15"
  Data Type Conversion15/1 -> Bus Creator/16  "e16"
  Data Type Conversion16/1 -> Bus Creator/17  "e17"
  Data Type Conversion17/1 -> Bus Creator/18  "e18"
  Data Type Conversion18/1 -> Bus Creator/19  "e19"
  Data Type Conversion19/1 -> Bus Creator/20  "e20"
  Data Type Conversion20/1 -> Bus Creator/21  "e21"
  Data Type Conversion21/1 -> Bus Creator/22  "e22"
  Data Type Conversion22/1 -> Bus Creator/23  "e23"
  Data Type Conversion23/1 -> Bus Creator/24  "e24"
  Constant/1 -> Data Type Conversion24/1, Data Type Conversion25/1, Data Type Conversion26/1, Data Type Conversion27/1, Data Type Conversion28/1, Data Type Conversion29/1, Data Type Conversion23/1, Data Type Conversion22/1, Data Type Conversion21/1, Data Type Conversion20/1, Data Type Conversion19/1, Data Type Conversion18/1, Data Type Conversion17/1, Data Type Conversion16/1, Data Type Conversion15/1, Data Type Conversion14/1, Data Type Conversion13/1, Data Type Conversion12/1, Data Type Conversion11/1, Data Type Conversion10/1, Data Type Conversion9/1, Data Type Conversion8/1, Data Type Conversion7/1, Data Type Conversion6/1, Data Type Conversion5/1, Data Type Conversion4/1, Data Type Conversion3/1, Data Type Conversion2/1, Data Type Conversion1/1, Data Type Conversion/1
  Data Type Conversion24/1 -> Bus Creator/25  "e25"
  Data Type Conversion25/1 -> Bus Creator/26  "e26"
  Data Type Conversion26/1 -> Bus Creator/27  "e27"
  Data Type Conversion27/1 -> Bus Creator/28  "e28"
  Data Type Conversion28/1 -> Bus Creator/29  "e29"
  Data Type Conversion29/1 -> Bus Creator/30  "e30"

== system PX4_Run_Mode_R2016b/CONTROLLER/Outer Control Loop/IMP Bus ==
  Bus Creator : BusCreator  Inputs=9
  Constant : Constant  Value=0  SampleTime=Ts
  Data Type Conversion{,1..8} (9 alike) : DataTypeConversion  OutDataTypeStr=single
  IMP_OUT : Outport
  wires:
  Bus Creator/1 -> IMP_OUT/1
  Data Type Conversion/1 -> Bus Creator/1  "Vx1"
  Data Type Conversion1/1 -> Bus Creator/2  "Vx2"
  Data Type Conversion2/1 -> Bus Creator/3  "Uxv"
  Data Type Conversion3/1 -> Bus Creator/4  "Vy1"
  Data Type Conversion4/1 -> Bus Creator/5  "Vy2"
  Data Type Conversion5/1 -> Bus Creator/6  "Uyv"
  Constant/1 -> Data Type Conversion6/1, Data Type Conversion7/1, Data Type Conversion8/1, Data Type Conversion5/1, Data Type Conversion4/1, Data Type Conversion3/1, Data Type Conversion2/1, Data Type Conversion1/1, Data Type Conversion/1
  Data Type Conversion6/1 -> Bus Creator/7  "Vz1"
  Data Type Conversion7/1 -> Bus Creator/8  "Vz2"
  Data Type Conversion8/1 -> Bus Creator/9  "Uzv"

== system PX4_Run_Mode_R2016b/CONTROLLER/Outer Control Loop/Thrust Control ==
  ERROR_IN : Inport
  TARGET : Inport  Port=2
  ESTIMATED_STATE_IN : Inport  Port=3
  SYSTEM_MODE_IN : Inport  Port=4
  Add : Sum  Inputs=-+
  Add2 : Sum  Inputs=-+
  Add5 : Sum
  Bus Assignment : BusAssignment  AssignedSignals=e26,e27,e28,e29,e30
  Bus Selector1 : BusSelector  OutputSignals=T_Z
  Bus Selector2 : BusSelector  OutputSignals=ARM_CMD,AUTO_FLIGHT,SEMI_AUTO_FLIGHT
  Bus Selector3 : BusSelector  OutputSignals=z,w
  Constant1 : Constant  Commented=on  Value=C24  SampleTime=Ts
  Constant2 : Constant  Value=-12.5  OutDataTypeStr=single
  Logical Operator : Logic  IconShape=distinctive  AllPortsSameDT=off  OutDataTypeStr=boolean
  Logical Operator1 : Logic  Operator=NOT  IconShape=distinctive  AllPortsSameDT=off  OutDataTypeStr=boolean
  Logical Operator2 : Logic  Operator=OR  IconShape=distinctive  AllPortsSameDT=off  OutDataTypeStr=boolean
  MATLAB Function2 : MATLAB Function  TreatAsAtomicUnit=on
  PID Controller : simulink/Continuous/PID Controller  Controller=PID  TimeDomain=Discrete-time  SampleTime=Ts  IntegratorMethod=Forward Euler  FilterMethod=Forward Euler  Form=Parallel  UseFilter=on  ControllerParametersSource=internal  P=2.0  I=0.9  D=0  N=100  InitialConditionSource=internal  InitialConditionForIntegrator=0  InitialConditionForFilter=0  ExternalReset=level  LimitOutput=off  UpperSaturationLimit=inf  LowerSaturationLimit=-inf  LinearizeAsGain=on  AntiWindupMode=none  Kb=1  TrackingMode=off  Kt=1  PParamMin=[]  PParamMax=[]  PParamDataTypeStr=single  IParamMin=[]  IParamMax=[]  IParamDataTypeStr=single  DParamMin=[]  DParamMax=[]  DParamDataTypeStr=single  NParamMin=[]  NParamMax=[]  NParamDataTypeStr=single  KbParamMin=[]  KbParamMax=[]  KtParamMin=[]  KtParamMax=[]  POutMin=[]  POutMax=[]  POutDataTypeStr=single  PGainOutDataTypeStr=single  PProdOutDataTypeStr=single  IOutMin=[]  IOutMax=[]  IOutDataTypeStr=single  IGainOutDataTypeStr=single  IProdOutDataTypeStr=single  DOutMin=[]  DOutMax=[]  DOutDataTypeStr=single  DGainOutDataTypeStr=single  DProdOutDataTypeStr=single  NOutMin=[]  NOutMax=[]  NOutDataTypeStr=single  NGainOutDataTypeStr=single  NProdOutDataTypeStr=single  KbOutMin=[]  KbOutMax=[]  KtOutMin=[]  KtOutMax=[]  IntegratorOutMin=[]  IntegratorOutMax=[]  IntegratorOutDataTypeStr=single  FilterOutMin=[]  FilterOutMax=[]  FilterOutDataTypeStr=single  SumOutMin=[]  SumOutMax=[]  SumOutDataTypeStr=single  SumI1OutMin=[]  SumI1OutMax=[]  SumI2OutMin=[]  SumI2OutMax=[]  SumI3OutMin=[]  SumI3OutMax=[]  SumDOutMin=[]  SumDOutMax=[]  SumDOutDataTypeStr=single  SumAccumDataTypeStr=single  SumDAccumDataTypeStr=single  SaturationOutMin=[]  SaturationOutMax=[]  IntegratorContinuousStateAttributes=''  IntegratorStateMustResolveToSignalObject=off  IntegratorRTWStateStorageClass=Auto  FilterContinuousStateAttributes=''  FilterStateMustResolveToSignalObject=off  FilterRTWStateStorageClass=Auto  DifferentiatorICPrevScaledInput=0  DifferentiatorOutMin=[]  DifferentiatorOutMax=[]
  PID Controller1 : simulink/Continuous/PID Controller  Controller=PID  TimeDomain=Discrete-time  SampleTime=Ts  IntegratorMethod=Forward Euler  FilterMethod=Forward Euler  Form=Parallel  UseFilter=on  ControllerParametersSource=internal  P=0.4  I=0  D=0  N=100  InitialConditionSource=internal  InitialConditionForIntegrator=0  InitialConditionForFilter=0  ExternalReset=none  LimitOutput=on  UpperSaturationLimit=0.33  LowerSaturationLimit=-0.33  LinearizeAsGain=on  AntiWindupMode=none  Kb=1  TrackingMode=off  Kt=1  PParamMin=[]  PParamMax=[]  IParamMin=[]  IParamMax=[]  DParamMin=[]  DParamMax=[]  NParamMin=[]  NParamMax=[]  KbParamMin=[]  KbParamMax=[]  KtParamMin=[]  KtParamMax=[]  POutMin=[]  POutMax=[]  IOutMin=[]  IOutMax=[]  DOutMin=[]  DOutMax=[]  NOutMin=[]  NOutMax=[]  KbOutMin=[]  KbOutMax=[]  KtOutMin=[]  KtOutMax=[]  IntegratorOutMin=[]  IntegratorOutMax=[]  FilterOutMin=[]  FilterOutMax=[]  SumOutMin=[]  SumOutMax=[]  SumI1OutMin=[]  SumI1OutMax=[]  SumI2OutMin=[]  SumI2OutMax=[]  SumI3OutMin=[]  SumI3OutMax=[]  SumDOutMin=[]  SumDOutMax=[]  SaturationOutMin=[]  SaturationOutMax=[]  IntegratorContinuousStateAttributes=''  IntegratorStateMustResolveToSignalObject=off  IntegratorRTWStateStorageClass=Auto  FilterContinuousStateAttributes=''  FilterStateMustResolveToSignalObject=off  FilterRTWStateStorageClass=Auto  DifferentiatorICPrevScaledInput=0  DifferentiatorOutMin=[]  DifferentiatorOutMax=[]
  U Z : Outport
  ERROR_OUT : Outport  Port=2
  wires:
  ESTIMATED_STATE_IN/1 -> Bus Selector3/1
  TARGET/1 -> Bus Selector1/1
  Bus Assignment/1 -> ERROR_OUT/1
  ERROR_IN/1 -> Bus Assignment/1
  SYSTEM_MODE_IN/1 -> Bus Selector2/1
  Bus Selector2/1 -> Logical Operator/1  "<ARM_CMD>"
  Logical Operator/1 -> Logical Operator1/1
  Logical Operator1/1 -> PID Controller/2
  Logical Operator2/1 -> Logical Operator/2
  Bus Selector2/2 -> Logical Operator2/1  "<AUTO_FLIGHT>"
  Bus Selector2/3 -> Logical Operator2/2  "<SEMI_AUTO_FLIGHT>"
  Bus Selector3/2 -> Add/1  "<w>"
  Bus Selector3/1 -> Add2/1  "<z>"
  PID Controller/1 -> Bus Assignment/4, Add5/1
  Add/1 -> Bus Assignment/3, PID Controller/1
  Bus Selector1/1 -> MATLAB Function2/1(T_z)  "<T_Z>"
  Add2/1 -> PID Controller1/1
  Add5/1 -> Bus Assignment/6, U Z/1
  Constant2/1 -> Bus Assignment/5, Add5/2
  MATLAB Function2/1(Z_Vel_Ref) -> Add2/2
  PID Controller1/1 -> Add/2, Bus Assignment/2
